simulink model "Q8a_Active_Cell_Balancing11"  (R2019a)
settings: Solver=daessc  StartTime=0.0  StopTime=120  RelTol=1e-3
undefined symbols (not defined in the file): Ion, Lithium
libraries: powerlib x15, electricdrivelib x2, powerlib_meascontrol x1
settings Model: Creator=harsh  LastModifiedBy=VIJAYPRASATH
settings DebuggingCC: UnconnectedInputMsg=none  UnconnectedOutputMsg=none  UnconnectedLineMsg=none
settings ModelReferenceCC: EnableRefExpFcnMdlSchedulingChecks=off
settings RTWCC: Description=Generic Real-Time Target

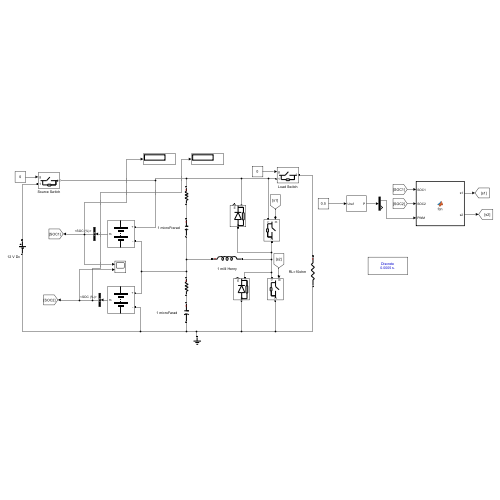
[thumbnail: Simulink's stored preview of the top-level diagram]
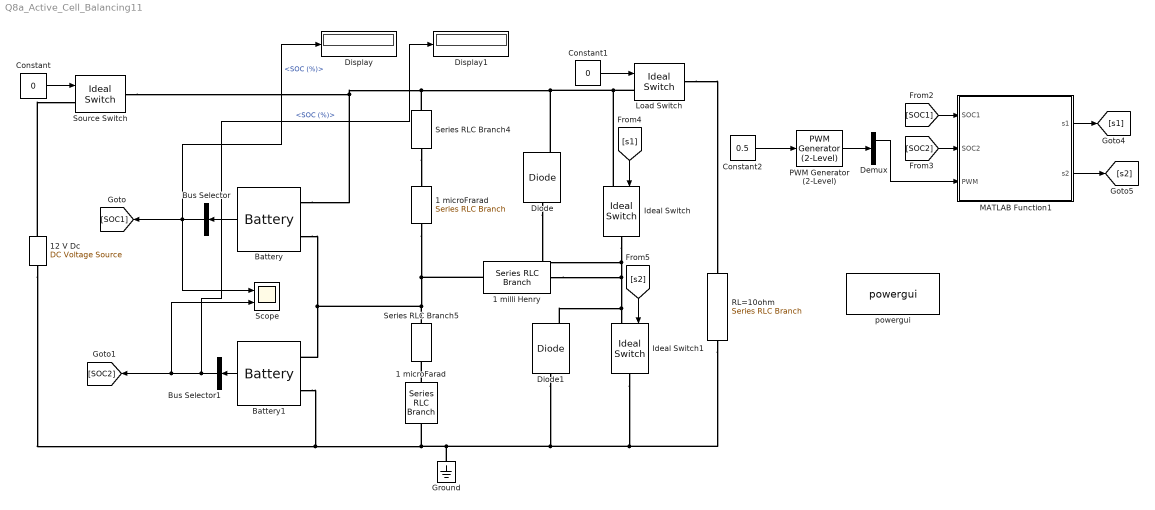
== system Q8a_Active_Cell_Balancing11 ==
  1 microFarad : powerlib/Elements/Series RLC Branch  LConnTagsString=__new0  RConnTagsString=__new0  BranchType=C  Resistance=1  Inductance=1e-3  SetiL0=off  InitialCurrent=0  Capacitance=1e-6  Setx0=off  InitialVoltage=0  Measurements=None
  1 microFrarad : powerlib/Elements/Series RLC Branch  LConnTagsString=__new0  RConnTagsString=__new0  BranchType=C  Resistance=1  Inductance=1e-3  SetiL0=off  InitialCurrent=0  Capacitance=1e-6  Setx0=off  InitialVoltage=0  Measurements=None
  1 milli Henry : powerlib/Elements/Series RLC Branch  LConnTagsString=__new0  RConnTagsString=__new0  BranchType=L  Resistance=1  Inductance=1e-3  SetiL0=off  InitialCurrent=0  Capacitance=1e-6  Setx0=off  InitialVoltage=0  Measurements=None
  "12 V Dc                 " : powerlib/Electrical Sources/DC Voltage Source  Amplitude=12  Measurements=None
  Battery : electricdrivelib/Extra Sources/Battery  BatType=Lithium-Ion  NomV=3.7  NomQ=5.4  SOC=50  Batt_Tr=30  PresetModel=on  MaxQ=5.4  MinV=2.775  FullV=4.3068  Dis_rate=2.3478  R=0.0068519  Normal_OP=4.8835  expZone="[3.9974      0.2653]"
  Battery1 : electricdrivelib/Extra Sources/Battery  BatType=Lithium-Ion  NomV=3.7  NomQ=5.4  SOC=30  Batt_Tr=30  PresetModel=on  MaxQ=5.4  MinV=2.775  FullV=4.3068  Dis_rate=2.3478  R=0.0068519  Normal_OP=4.8835  expZone="[3.9974      0.2653]"
  Bus Selector : BusSelector  OutputSignals=SOC (%)
  Bus Selector1 : BusSelector  OutputSignals=SOC (%)
  Constant : Constant  Value=0
  Constant1 : Constant  Value=0
  Constant2 : Constant  Value=0.5
  Demux : Demux  Outputs=2
  Diode : powerlib/Power Electronics/Diode  Ron=0.001  Lon=0  Vf=0.8  IC=0  UseSnubber=0  Rs=500  Cs=250e-9  Measurements=on
  Diode1 : powerlib/Power Electronics/Diode  Ron=0.001  Lon=0  Vf=0.8  IC=0  UseSnubber=0  Rs=500  Cs=250e-9  Measurements=on
  Display : Display
  Display1 : Display
  Ground : powerlib/Elements/Ground  LConnTagsString=a
  Ideal Switch : powerlib/Power Electronics/Ideal Switch  Ron=0.001  Lon=0  IC=0  Rs=1e5  Cs=inf  Measurements=off
  Ideal Switch1 : powerlib/Power Electronics/Ideal Switch  Ron=0.001  Lon=0  IC=0  Rs=1e5  Cs=inf  Measurements=off
  Load Switch : powerlib/Power Electronics/Ideal Switch  Ron=0.001  Lon=0  IC=0  Rs=1e5  Cs=inf  Measurements=off
  MATLAB Function1 : MATLAB Function  TreatAsAtomicUnit=on
  PWM Generator (2-Level) : powerlib_meascontrol/Pulse & Signal Generators/PWM Generator (2-Level)  ModulatorType=Single-phase half-bridge (2 pulses)  ModulatorMode=Unsynchronized  Fc=500  Pc=0  nF=27  MinMax="[ -1  1 ]"  SamplingTechnique=Natural  ModulatingSignals=off  m=0.8  Freq=60  Phase=0  Ts=0  ShowCarrierOutport=off
  RL=10ohm : powerlib/Elements/Series RLC Branch  LConnTagsString=__new0  RConnTagsString=__new0  BranchType=R  Resistance=10  Inductance=1e-3  SetiL0=off  InitialCurrent=0  Capacitance=1e-6  Setx0=off  InitialVoltage=0  Measurements=None
  Scope : Scope  NumInputPorts=2
  Series RLC Branch4 : powerlib/Elements/Series RLC Branch  LConnTagsString=__new0  RConnTagsString=__new0  BranchType=R  Resistance=0.1  Inductance=1e-3  SetiL0=off  InitialCurrent=0  Capacitance=1e-6  Setx0=off  InitialVoltage=0  Measurements=None
  Series RLC Branch5 : powerlib/Elements/Series RLC Branch  LConnTagsString=__new0  RConnTagsString=__new0  BranchType=R  Resistance=0.1  Inductance=1e-3  SetiL0=off  InitialCurrent=0  Capacitance=1e-6  Setx0=off  InitialVoltage=0  Measurements=None
  Source Switch : powerlib/Power Electronics/Ideal Switch  Ron=0.001  Lon=0  IC=0  Rs=1e5  Cs=inf  Measurements=off
  powergui : powerlib/powergui  Priority=1  SimulationMode=Discrete  SampleTime=50e-5  frequency=60  Iterations=50  frequencyindice=0  Pbase=100e6  ErrMax=1e-4  UnitsV=kV  UnitsW=MW  buscounter=0  FunctionMessages=off  echomessages=off  EnableUseOfTLC=off  CurrentSourceSwitches=off  DisableSnubberDevices=off  DisableRonSwitches=off  DisableVfSwitches=off  DisplayEquations=off  AutomaticDiscreteSolvers=off  SolverType=Tustin/Backward Euler (TBE)  Interpol=off  ExternalGateDelay=off  methode=off  Ts=100  x0status=blocks  SPID=on  SwTol=0  HookPort=off  NonlinearTolerance=1e-4  nMaxIteration=100  ContinueOnMaxIteration=off  RestoreLinks=warning  ResistiveCurrentMeasurement=off  Frange=[0:2:500]  Ylog=off  Xlog=on  ShowGrid=off  save=off  variable=ZData  structure=0  ZoomFFT=off  StartTime=0.0  cycles=1  DisplayStyle=1  fundamental=60  FreqAxis=off  MaxFrequency=1000  frequencyindicesteady=1  RmsSteady=1  display=off
  wires:
  Battery/1 -> Bus Selector/1
  Bus Selector/1 -> Scope/1, Display/1, [SOC1]  "<SOC (%)>"
  [s1] -> Ideal Switch/1
  [s2] -> Ideal Switch1/1
  Battery1/1 -> Bus Selector1/1
  Bus Selector1/1 -> Scope/2, [SOC2], Display1/1  "<SOC (%)>"
  Constant/1 -> Source Switch/1
  Constant1/1 -> Load Switch/1
  Constant2/1 -> PWM Generator (2-Level)/1
  [SOC1] -> MATLAB Function1/1(SOC1)
  [SOC2] -> MATLAB Function1/2(SOC2)
  MATLAB Function1/1(s1) -> [s1]
  MATLAB Function1/2(s2) -> [s2]
  PWM Generator (2-Level)/1 -> Demux/1
  Demux/1 -> MATLAB Function1/3(PWM)
  connections:
  Battery/LConn2 -- Battery1/LConn1 -- 1 milli Henry/LConn1 -- 1 microFrarad/RConn1 -- Series RLC Branch5/LConn1
  Ideal Switch/RConn1 -- Ideal Switch1/LConn1 -- Diode1/RConn1 -- 1 milli Henry/RConn1 -- Diode/LConn1
  "12 V Dc                 "/LConn1 -- Ground/LConn1 -- Diode1/LConn1 -- Ideal Switch1/RConn1 -- RL=10ohm/RConn1 -- 1 microFarad/RConn1 -- Battery1/LConn2
  Load Switch/LConn1 -- Ideal Switch/LConn1 -- Battery/LConn1 -- Source Switch/RConn1 -- Series RLC Branch4/LConn1 -- Diode/RConn1
  "12 V Dc                 "/RConn1 -- Source Switch/LConn1
  Load Switch/RConn1 -- RL=10ohm/LConn1
  Series RLC Branch4/RConn1 -- 1 microFrarad/LConn1
  1 microFarad/LConn1 -- Series RLC Branch5/RConn1

== matlab function Q8a_Active_Cell_Balancing11/MATLAB Function1 ==
  data: SOC1 input; s1 output; SOC2 input; PWM input; s2 output
function [s1,s2] = fcn(SOC1,SOC2,PWM)
if SOC2<SOC1
    s1=PWM;
    s2=0;
elseif SOC1<SOC2
    s1=0;
    s2=PWM;
else 
    s1=0;
    s2=0;
end
